simulink model "sim_ls_mpc"  (R2022b)
settings: Solver=VariableStepAuto  StartTime=0.0  StopTime=4  RelTol=1e-3
values from neighbouring files (symbols this model uses):
  lbu_sim = repmat(model.input_constraints(:,1),N,1)    [srbd_ocp.m]
  nx = 7    [srbd_model.m]    (also in srbd_ocp.m = model.nx)
  ubu_sim = repmat(model.input_constraints(:,2),N,1)    [srbd_ocp.m]
  y_ref = [Qc,zeros(nx,nu);zeros(nu,nx),Rc]*[xref;0;0;0]    [srbd_ocp.m]
  y_ref_sim = repmat(y_ref,N-1,1)    [srbd_ocp.m]
settings Model: Creator=papaveneti  LastModifiedBy=papaveneti

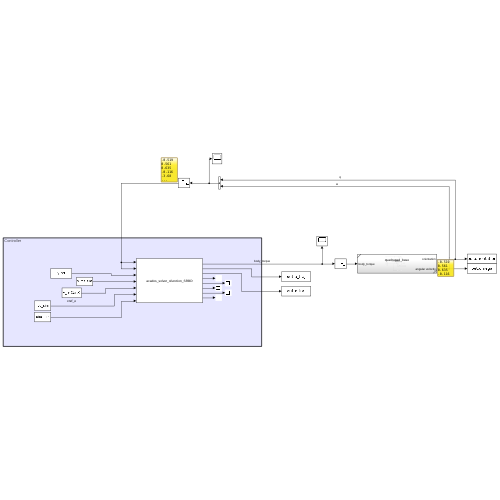
[thumbnail: Simulink's stored preview of the top-level diagram]
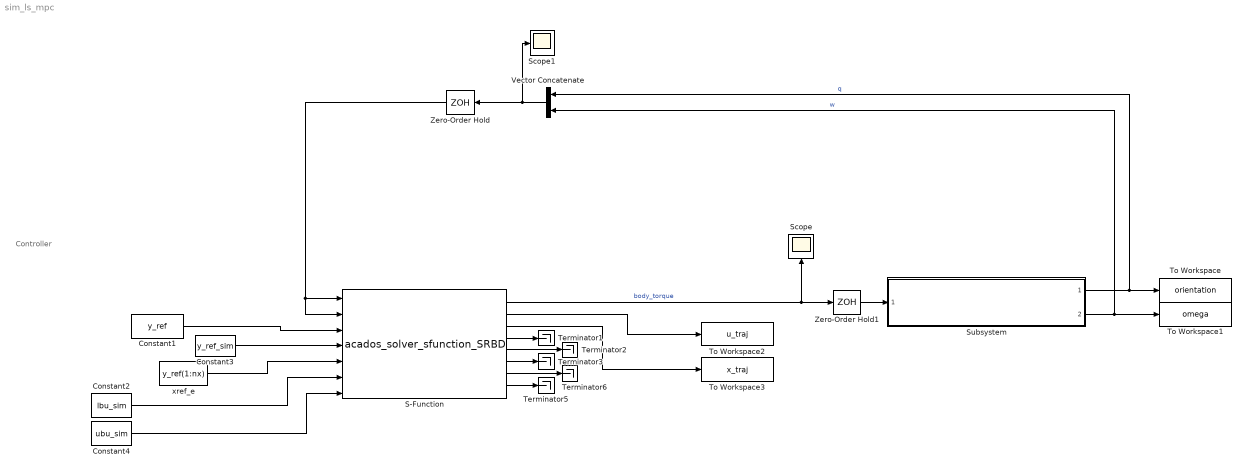
== system sim_ls_mpc ==
  note: Controller
  Constant1 : Constant  Value=y_ref
  Constant2 : Constant  Value=lbu_sim
  Constant3 : Constant  Value=y_ref_sim
  Constant4 : Constant  Value=ubu_sim
  S-Function : S-Function  FunctionName=acados_solver_sfunction_SRBD  SFunctionDeploymentMode=off  EnableBusSupport=off
  Scope : Scope
  Scope1 : Scope
  Subsystem : Subsystem  ReferencedSubsystem=quadruped_base
  Terminator{1..3,5..6} (5 alike) : Terminator
  To Workspace : ToWorkspace  VariableName=orientation  SaveFormat=Timeseries  SampleTime=-1
  To Workspace1 : ToWorkspace  VariableName=omega  SaveFormat=Timeseries  SampleTime=-1
  To Workspace2 : ToWorkspace  VariableName=u_traj  SaveFormat=Timeseries  SampleTime=-1
  To Workspace3 : ToWorkspace  VariableName=x_traj  SaveFormat=Timeseries  SampleTime=-1
  Vector Concatenate : Concatenate
  Zero-Order Hold : ZeroOrderHold  SampleTime=0.001
  Zero-Order Hold1 : ZeroOrderHold  SampleTime=0.001
  xref_e : Constant  Value=y_ref(1:nx)
  wires:
  S-Function/1 -> Zero-Order Hold1/1, Scope/1  "body_torque"
  Subsystem/2 -> Vector Concatenate/2, To Workspace1/1  "w"
  Subsystem/1 -> Vector Concatenate/1, To Workspace/1  "q"
  Constant1/1 -> S-Function/3
  xref_e/1 -> S-Function/5
  Constant3/1 -> S-Function/4
  Constant2/1 -> S-Function/6
  Constant4/1 -> S-Function/7
  S-Function/2 -> To Workspace2/1
  S-Function/3 -> To Workspace3/1
  S-Function/4 -> Terminator1/1
  S-Function/5 -> Terminator2/1
  S-Function/6 -> Terminator3/1
  S-Function/8 -> Terminator5/1
  S-Function/7 -> Terminator6/1
  Vector Concatenate/1 -> Scope1/1, Zero-Order Hold/1
  Zero-Order Hold/1 -> S-Function/2, S-Function/1
  Zero-Order Hold1/1 -> Subsystem/1
